simulink model "fully_dependent_mode"  (R2018b)
settings: Solver=VariableStepAuto  StartTime=0.0  StopTime=140.0  RelTol=1e-3
settings Model: Creator=gautam  LastModifiedBy=gautam

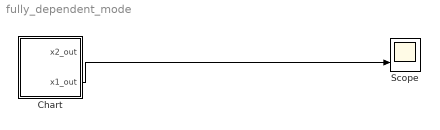
== system fully_dependent_mode ==
  Chart : Stateflow chart  TreatAsAtomicUnit=on
  Scope : Scope  NumInputPorts=2
  wires:
  Chart/2(x1_out) -> Scope/2

== stateflow chart fully_dependent_mode/Chart ==
  settings: updateMethod=CONTINUOUS
  state Off1
    du:
    x1_dot = -0.01*x1;
    x1 = x2;
    x2 = x4 + x3;
    x4 = x5;
  data: x2_out output double; x1_out output double; x2 local; x1 local
  data x2 settings: updateMethod=SF_CONTINUOUS_TIME_DATA
  data x1 settings: updateMethod=SF_CONTINUOUS_TIME_DATA
